simulink model "receiver"  (R2020b)
settings: Solver=VariableStepAuto  StartTime=0.0  StopTime=20  RelTol=1e-3
undefined symbols (not defined in the file): Fs, ip, usb
libraries: dspmlti4 x2, plutoradiolib x1, dspsnks4 x1
settings Model: Creator=hp  LastModifiedBy=JYLIU
settings SFSimCC: CustomCodeUndefinedFunction=UseInterfaceOnly

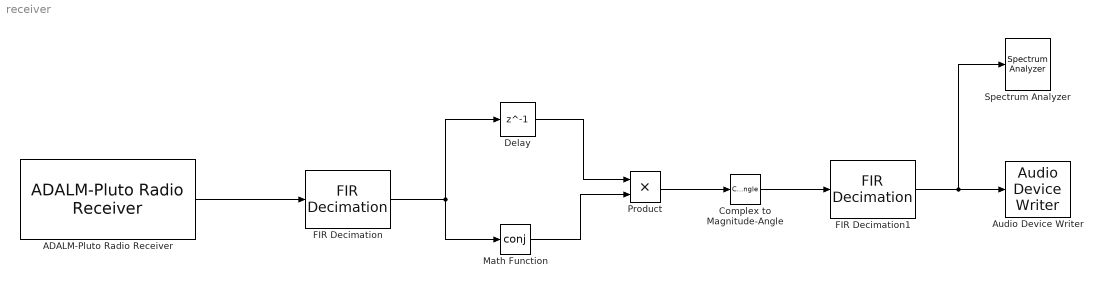
== system receiver ==
  ADALM-Pluto Radio Receiver : plutoradiolib/ADALM-Pluto Radio Receiver  RadioID=usb:0  uri=ip:10.0.0.200  CenterFrequencySource=Dialog  CenterFrequency=91.6e6  GainSource=AGC Slow Attack  GainSourceBlock=AGC Slow Attack  Gain=10  ChannelMapping=1  BasebandSampleRate=2.4e6  OutputDataType=double  SamplesPerFrame=32768  OverflowOutputPort=off  EnableBurstMode=off  NumFramesInBurst=1  ShowAdvancedProperties=off  UseCustomFilter=off  filtPathRates=[737280000 11520000 3840000 1920000 960000 240000]  filtCoefficients=[-192 82 85 -215 228 -102 -110 290 -318 145 160 -426 471 -215 -238 633 -697 318 349 -923 1009 -457 -498 1309 -1423 640 693 -1812 1959 -876 -945 2458 -2647 1180 1268 -3290 3534 -1572 -1688 4375 -4698 2091 2247 -5836 6284 -2807 -3031 7918 -8588 3870 4225 -11182 12324 -5662 -6330 17255 -19735 9507 11312 -33568 43355 -25227 -42139 305542 305542 -42139 -25227 43355 -33568 11312 9507 -19735 17255 -6330 -5662 12324 -11182 4225 3870 -8588 7918 -3031 -2807 6284 -5836 2247 2091 -4698 4375 -1688 -1572 3534 -3290 1268 1180 -2647 2458 -945 -876 1959 -1812 693 640 -1423 1309 -498 -457 1009 -923 349 318 -697 633 -238 -215 471 -426 160 145 -318 290 -110 -102 228 -215 85 82 -192]  filtCoefficientSize=128  filtDecimInterpFactor=4  filtGain=-12  filtRFBandwidth=18000000  filterConfigStruct=struct()  EnableQuadratureCorrection=on  EnableRFDCCorrection=on  EnableBasebandDCCorrection=on  FrequencyCorrection=0  OverrideSampleTime=off  SampleTime=0.02  DataTimeout=Inf  ENSMPinControlMode=None  BISTLoopbackMode=Disabled  BISTToneInject=Disabled  BISTSignalGen=PRBS  BISTToneFreq=Fs/32  BISTToneLevel=0
      settings: SourceProductBaseCode=PLUTO
  Audio Device Writer : dspsnks4/Audio Device Writer  Driver=DirectSound  Device=Default  InheritSampleRate=on  SampleRate=44100  BitDepth=16-bit integer  BufferSize=4096  NumBuffers=10  DefaultOutputChannelMapping=on  OutputChannelMapping=1:2  OutputNumUnderrunSamples=off  DriverIdx=1  DeviceWarnFlag=''
  Complex to Magnitude-Angle : ComplexToMagnitudeAngle  Output=Angle
  Delay : Delay  DelayLength=1  InputProcessing=Columns as channels (frame based)
  FIR Decimation : dspmlti4/FIR Decimation  FilterSource=Dialog parameters  h=firpm(50,[0 120e3 240e3 (2.4e6/2)]/(2.4e6/2), [1 1 0 0], [1 1],20)  D=10  filtStruct=Direct form  FilterObject=FDECIM  InputProcessing=Columns as channels (frame based)  framing=Allow multirate processing  inputOffset=0  outputBufInitCond=0  roundingMode=Floor  overflowMode=off  firstCoeffDataTypeStr=Inherit: Same word length as input  firstCoeffMin=[]  firstCoeffMax=[]  firstCoeffLastDataTypeStr=Inherit: Same word length as input  outputDataTypeStr=Inherit: Same as accumulator  outputMin=[]  outputMax=[]  outputLastDataTypeStr=Inherit: Same as accumulator
  FIR Decimation1 : dspmlti4/FIR Decimation  FilterSource=Dialog parameters  h=firpm(100,[0 15e3 20e3 (240e3/2)]/(240e3/2), [1 1 0 0], [1 1],20)  D=5  filtStruct=Direct form  FilterObject=FDECIM  InputProcessing=Columns as channels (frame based)  framing=Allow multirate processing  inputOffset=0  outputBufInitCond=0  roundingMode=Floor  overflowMode=off  firstCoeffDataTypeStr=Inherit: Same word length as input  firstCoeffMin=[]  firstCoeffMax=[]  firstCoeffLastDataTypeStr=Inherit: Same word length as input  outputDataTypeStr=Inherit: Same as accumulator  outputMin=[]  outputMax=[]  outputLastDataTypeStr=Inherit: Same as accumulator
  Math Function : Math  Operator=conj  SignedPower=on  SaturateOnIntegerOverflow=on
  Product : Product
  Spectrum Analyzer : SpectrumAnalyzer
  wires:
  ADALM-Pluto Radio Receiver/1 -> FIR Decimation/1
  FIR Decimation/1 -> Math Function/1, Delay/1
  Delay/1 -> Product/1
  Math Function/1 -> Product/2
  Product/1 -> Complex to Magnitude-Angle/1
  Complex to Magnitude-Angle/1 -> FIR Decimation1/1
  FIR Decimation1/1 -> Spectrum Analyzer/1, Audio Device Writer/1
